simulink model "QuadRotor_Simulink_LQT"  (R2021b)
settings: Solver=ode23tb  StartTime=0.0  StopTime=30  RelTol=1e-3
values from neighbouring files (symbols this model uses):
  A = qrs.LinearPlantModel.A    [ControllerDev.m]    (also in ControllerDev_Aksland.m)
  B = qrs.LinearPlantModel.B    [ControllerDev.m]    (also in ControllerDev_Aksland.m)
  C = eye(size(A))    [ControllerDev.m]    (also in ControllerDev_Aksland.m = qrs.LinearPlantModel.C)
  D = zeros(size(C,1),size(B,2))    [ControllerDev.m]    (also in ControllerDev_Aksland.m)
  K = zeros(size(B,2), size(A,1), numel(t))    [ControllerDev.m]    (also in ControllerDev_Aksland.m = lqr(A,B,Q,R))
  Kcol = reshape(K,size(K,1)*size(K,2),size(K,3), 1)    [ControllerDev.m]
  nu_0 = nu(end,:)'    [ControllerDev.m]
  Q = eye(size(C,1))    [ControllerDev.m]    (also in ControllerDev_Aksland.m = eye(size(A)))
  R = rho*eye(size(B,2))    [ControllerDev.m]    (also in ControllerDev_Aksland.m = eye(size(B,2)))
  Tf = Times(end)    [ControllerDev.m]
undefined symbols (not defined in the file or in its folder): Kstatic, QR_Object, tk
libraries: simulink_extras x1, uavutilslib x1
settings Model: Creator=renkert2  LastModifiedBy=renkert2
settings SolverCC: AlgebraicLoopSolver=TrustRegion
settings DebuggingCC: SFMachineParentedDataDiag=warning

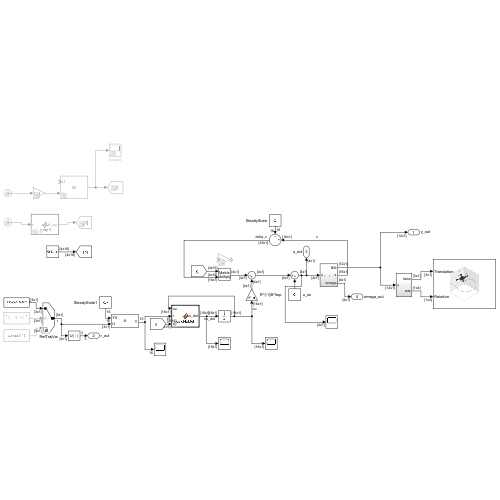
[thumbnail: Simulink's stored preview of the top-level diagram]
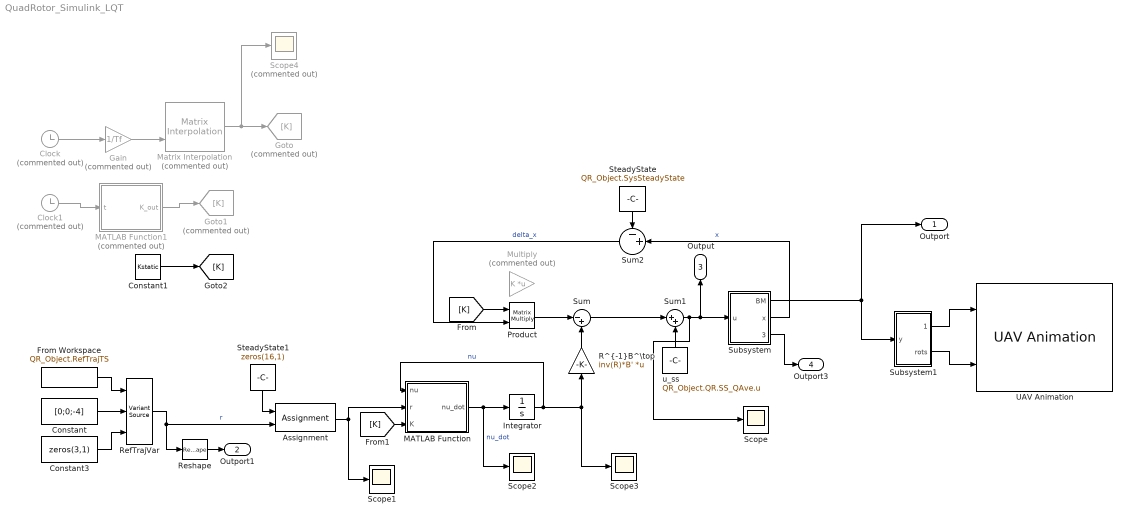
== system QuadRotor_Simulink_LQT ==
  Assignment : Assignment  DiagnosticForDimensions=Warning  IndexOptions=Index vector (dialog)  Indices=[5 6 7]  OutputSizes=1
  Clock : Clock  Commented=on
  Clock1 : Clock  Commented=on
  Constant : Constant  Value=[0;0;-4]
  Constant1 : Constant  Value=Kstatic
  Constant3 : Constant  Value=zeros(3,1)
  From Workspace : FromWorkspace  VariableName=QR_Object.RefTrajTS  OutputAfterFinalValue=Holding final value
  Gain : Gain  Commented=on  Gain=1/Tf
  Goto : Goto  Commented=on  GotoTag=K
  Goto1 : Goto  Commented=on  GotoTag=K
  Integrator : Integrator  InitialCondition=nu_0
  MATLAB Function : MATLAB Function  TreatAsAtomicUnit=on  mask{A=A, B=B, C=C, K=K, Q=Q}
  MATLAB Function1 : MATLAB Function  Commented=on  TreatAsAtomicUnit=on  mask{tk=tk, K=K, Kcol=Kcol}
  Matrix Interpolation : simulink_extras/Additional Lookup Tables/Matrix Interpolation  Commented=on  InterpMethod=Linear  ExtrapMethod=Clip  InterpolateDimension=1  TableData=K  SimulateUsing=Code generation
      settings: SourceProductBaseCode=SL
  Multiply : Gain  Commented=on  Gain=K  Multiplication=Matrix(K*u)
  Product : Product  Multiplication=Matrix(*)
  "R^{-1}B^\\top" : Gain  Gain=inv(R)*B'  Multiplication=Matrix(K*u)
  RefTrajVar : VariantSource  VariantControlMode=label  LabelModeActiveChoice=TimeSeries
  Reshape : Reshape
  Scope{,1..3} (4 alike) : Scope
  Scope4 : Scope  Commented=on
  SteadyState : Constant  Value=QR_Object.SysSteadyState
  SteadyState1 : Constant  Value=zeros(16,1)
  Subsystem : Subsystem
  Subsystem1 : Subsystem
  Sum : Sum  Inputs=|-+
  Sum1 : Sum  Inputs=|++
  Sum2 : Sum  Inputs=-+|
  UAV Animation : uavutilslib/UAV Animation  UAVType=Multirotor  UAVSize=1  InertialZDirection=Down  SampleTime=-1
      settings: SourceProductBaseCode=UV
  u_ss : Constant  Value=QR_Object.QR.SS_QAve.u  VectorParams1D=off
  Outport : Outport  SignalName=y_out
  Outport1 : Outport  Port=2  SignalName=r_out
  Output : Outport  Port=3  SignalName=u_out
  Outport3 : Outport  Port=4  SignalName=omega_out
  wires:
  From Workspace/1 -> RefTrajVar/1
  Reshape/1 -> Outport1/1
  Subsystem/1(BM) -> Subsystem1/1(y), Outport/1
  Constant/1 -> RefTrajVar/2
  RefTrajVar/1 -> Assignment/2, Reshape/1  "r"
  Subsystem/2(x) -> Sum2/2  "x"
  u_ss/1 -> Sum1/2
  Sum1/1 -> Scope/1, Subsystem/1(u), Output/1
  Subsystem/3(omega) -> Outport3/1
  Constant3/1 -> RefTrajVar/3
  SteadyState/1 -> Sum2/1
  Sum2/1 -> Product/2  "delta_x"
  Sum/1 -> Sum1/1
  "R^{-1}B^\\top"/1 -> Sum/2
  Integrator/1 -> MATLAB Function/1(nu), Scope3/1, "R^{-1}B^\\top"/1  "nu"
  MATLAB Function/1(nu_dot) -> Scope2/1, Integrator/1  "nu_dot"
  Subsystem1/1(trans) -> UAV Animation/1
  Subsystem1/2(rots) -> UAV Animation/2
  SteadyState1/1 -> Assignment/1
  Assignment/1 -> MATLAB Function/2(r), Scope1/1
  Product/1 -> Sum/1
  Clock/1 -> Gain/1
  Gain/1 -> Matrix Interpolation/2
  Matrix Interpolation/1 -> Scope4/1, Goto/1
  Clock1/1 -> MATLAB Function1/1(t)
  MATLAB Function1/1(K_out) -> Goto1/1
  [K] -> Product/1
  [K] -> MATLAB Function/3(K)
  Constant1/1 -> [K]

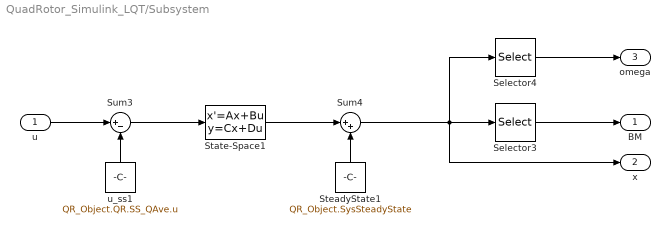
== system QuadRotor_Simulink_LQT/Subsystem ==
  u : Inport
  Selector3 : Selector  InputPortWidth=16  IndexOptions=Index vector (dialog)  Indices=5:16  OutputSizes=1
  Selector4 : Selector  InputPortWidth=16  IndexOptions=Index vector (dialog)  Indices=1:4  OutputSizes=1
  State-Space1 : StateSpace  A=A  B=B  C=C  D=D  InitialCondition=0
  SteadyState1 : Constant  Value=QR_Object.SysSteadyState
  Sum3 : Sum  Inputs=|+-
  Sum4 : Sum  Inputs=|++
  u_ss1 : Constant  Value=QR_Object.QR.SS_QAve.u  VectorParams1D=off
  BM : Outport
  x : Outport  Port=2
  omega : Outport  Port=3
  wires:
  Sum4/1 -> x/1, Selector4/1, Selector3/1
  u_ss1/1 -> Sum3/2
  State-Space1/1 -> Sum4/1
  SteadyState1/1 -> Sum4/2
  u/1 -> Sum3/1
  Selector3/1 -> BM/1
  Selector4/1 -> omega/1
  Sum3/1 -> State-Space1/1

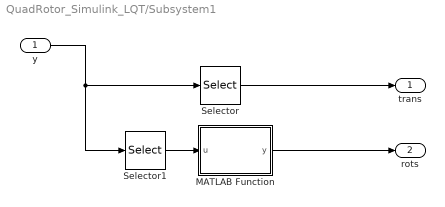
== system QuadRotor_Simulink_LQT/Subsystem1 ==
  y : Inport
  MATLAB Function : MATLAB Function  TreatAsAtomicUnit=on
  Selector : Selector  InputPortWidth=QR_Object.QR.BM.Nx  IndexOptions=Index vector (dialog)  Indices=QR_Object.QR.BM.I.x.p  OutputSizes=1
  Selector1 : Selector  InputPortWidth=QR_Object.QR.BM.Nx  IndexOptions=Index vector (dialog)  Indices=QR_Object.QR.BM.I.x.Theta  OutputSizes=1
  trans : Outport
  rots : Outport  Port=2
  wires:
  Selector/1 -> trans/1
  Selector1/1 -> MATLAB Function/1(u)
  y/1 -> Selector/1, Selector1/1
  MATLAB Function/1(y) -> rots/1

== matlab function QuadRotor_Simulink_LQT/Subsystem1/MATLAB Function ==
  data: u input; y output
function y = eul2quatMF(u)
    y = eul2quat([1 -1 1].*fliplr(u'),'ZYX');
end

== matlab function QuadRotor_Simulink_LQT/MATLAB Function ==
  data: nu input; r input; nu_dot output; A parameter; B parameter; C parameter; Q parameter; K input
function nu_dot  = calcNuDot(nu, r, A, B, C, Q, K)
nu_dot = ((A - B*K)'*nu + C'*Q*r);

== matlab function QuadRotor_Simulink_LQT/MATLAB Function1 ==
  data: t input; K_out output; tk parameter; Kcol parameter; K parameter
function K_out = InterpK(t, tk, Kcol, K)
K_out = reshape(interp1(tk',Kcol',t), size(K,1), size(K,2));
end
